simulink model "Guia_9_Ejercicio_4_simulink"  (R2016a)
settings: Solver=VariableStepAuto  StartTime=0.0  StopTime=8  RelTol=1e-3
values from neighbouring files (symbols this model uses):
  A = [ 0 1 0 ; 0 0 1; -1 -5 -6]    [Guia_9_Ejercicio_2.m]
  B = [0; 0 ; 1]    [Guia_9_Ejercicio_2.m]
  C = KCRAF * KCRRF * GRRF * GRAF    [ejercicio5guia8.m]
undefined symbols (not defined in the file or in its folder): D
settings Model: Creator=Abel  LastModifiedBy=Abel

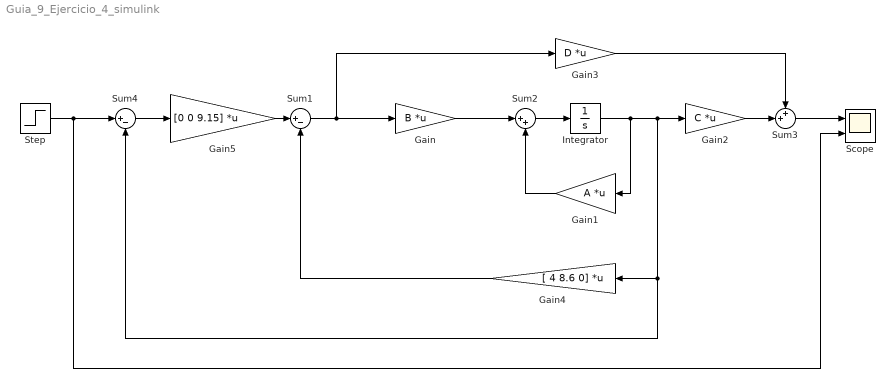
== system Guia_9_Ejercicio_4_simulink ==
  Gain : Gain  Gain=B  Multiplication=Matrix(K*u) (u vector)
  Gain1 : Gain  Gain=A  Multiplication=Matrix(K*u) (u vector)
  Gain2 : Gain  Gain=C  Multiplication=Matrix(K*u) (u vector)
  Gain3 : Gain  Gain=D  Multiplication=Matrix(K*u) (u vector)
  Gain4 : Gain  Gain=[ 4 8.6 0]  Multiplication=Matrix(K*u) (u vector)
  Gain5 : Gain  Gain=[0 0 9.15]  Multiplication=Matrix(K*u) (u vector)
  Integrator : Integrator
  Scope : Scope  NumInputPorts=2
  Step : Step  SampleTime=0
  Sum1 : Sum  Inputs=|+-
  Sum2 : Sum  Inputs=|++
  Sum3 : Sum  Inputs=++|
  Sum4 : Sum  Inputs=|+-
  wires:
  Sum1/1 -> Gain3/1, Gain/1
  Gain/1 -> Sum2/1
  Sum2/1 -> Integrator/1
  Gain1/1 -> Sum2/2
  Integrator/1 -> Sum4/2, Gain4/1, Gain2/1, Gain1/1
  Gain2/1 -> Sum3/2
  Gain3/1 -> Sum3/1
  Sum3/1 -> Scope/1
  Gain4/1 -> Sum1/2
  Gain5/1 -> Sum1/1
  Sum4/1 -> Gain5/1
  Step/1 -> Scope/2, Sum4/1
